simulink model "Product_TestGen3"  (R2017b)
settings: Solver=FixedStepDiscrete  StartTime=0.0  StopTime=10.0  RelTol=1e-3
undefined symbols (not defined in the file): Block_TestLib, enable
settings Model: Creator=ktrinh  LastModifiedBy=ktrinh
settings DebuggingCC: ParameterOverflowMsg=none

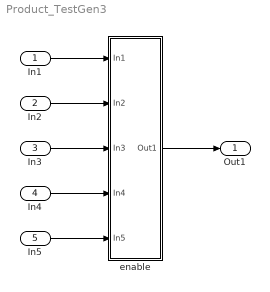
== system Product_TestGen3 ==
  In1 : Inport
  In2 : Inport  Port=2
  In3 : Inport  Port=3
  In4 : Inport  Port=4
  In5 : Inport  Port=5
  enable : Subsystem  AncestorBlock=Block_TestLib/enable
  Out1 : Outport
  wires:
  In1/1 -> enable/1(In1)
  In2/1 -> enable/2(In2)
  In3/1 -> enable/3(In3)
  In4/1 -> enable/4(In4)
  In5/1 -> enable/5(In5)
  enable/1(Out1) -> Out1/1

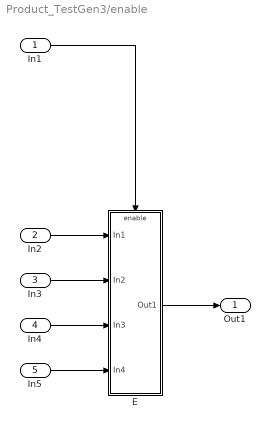
== system Product_TestGen3/enable ==
  In1 : Inport  OutDataTypeStr=boolean
  In2 : Inport  Port=2
  In3 : Inport  Port=3
  In4 : Inport  Port=4
  In5 : Inport  Port=5
  E : Subsystem  TreatAsAtomicUnit=on
  Out1 : Outport
  wires:
  In1/1 -> E/Enable
  In2/1 -> E/1(In1)
  In3/1 -> E/2(In2)
  In4/1 -> E/3(In3)
  In5/1 -> E/4(In4)
  E/1(Out1) -> Out1/1

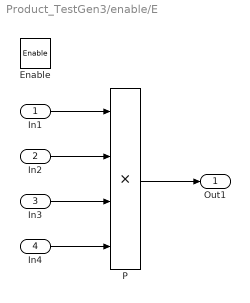
== system Product_TestGen3/enable/E ==
  In1 : Inport  OutDataTypeStr=int8  PortDimensions=1
  In2 : Inport  Port=2  OutDataTypeStr=int8  PortDimensions=1
  In3 : Inport  Port=3  OutDataTypeStr=int8  PortDimensions=1
  In4 : Inport  Port=4  OutDataTypeStr=int8  PortDimensions=1
  Enable : EnablePort
  P : Product  Inputs=4  OutDataTypeStr=int8
  Out1 : Outport
  wires:
  In1/1 -> P/1
  In2/1 -> P/2
  In3/1 -> P/3
  In4/1 -> P/4
  P/1 -> Out1/1
